simulink subsystem "Swerve_Drive_sub"  (R2023b)
settings: Solver=VariableStepAuto  StartTime=0.0  StopTime=10.0  RelTol=1e-3
undefined symbols (not defined in the file): Distance_BL_x, Distance_BL_y, Distance_BR_x, Distance_BR_y, Distance_FL_x, Distance_FL_y, Distance_FR_x, Distance_FR_y
libraries: Controls_Components_lib x8, simulink_extras x1
settings Model: Creator=ander  LastModifiedBy=ander

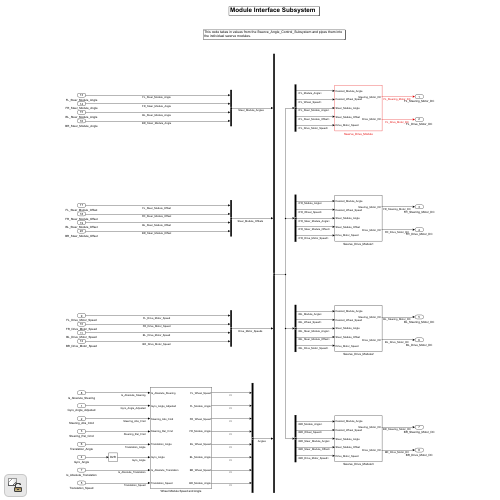
[thumbnail: Simulink's stored preview of the top-level diagram]
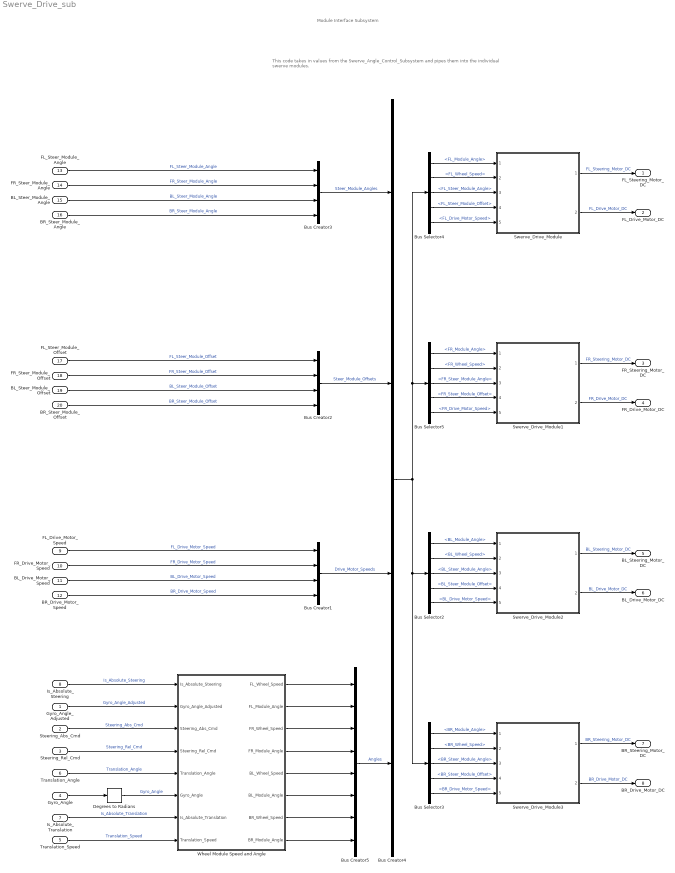
== system Swerve_Drive_sub ==
  note: This code takes in values from the Swerve_Angle_Control_Subsystem and pipes them into the individual swerve modules.
  note: Module Interface Subsystem
  Gyro_Angle_Adjusted : Inport
  Steering_Abs_Cmd : Inport  Port=2
  Steering_Rel_Cmd : Inport  Port=3
  Gyro_Angle : Inport  Port=4
  Translation_Speed : Inport  Port=5
  Translation_Angle : Inport  Port=6
  Is_Absolute_Translation : Inport  Port=7
  Is_Absolute_Steering : Inport  Port=8
  FL_Drive_Motor_Speed : Inport  Port=9
  FR_Drive_Motor_Speed : Inport  Port=10
  BL_Drive_Motor_Speed : Inport  Port=11
  BR_Drive_Motor_Speed : Inport  Port=12
  FL_Steer_Module_Angle : Inport  Port=13
  FR_Steer_Module_Angle : Inport  Port=14
  BL_Steer_Module_Angle : Inport  Port=15
  BR_Steer_Module_Angle : Inport  Port=16
  FL_Steer_Module_Offset : Inport  Port=17
  FR_Steer_Module_Offset : Inport  Port=18
  BL_Steer_Module_Offset : Inport  Port=19
  BR_Steer_Module_Offset : Inport  Port=20
  Bus Creator{1..4} (4 alike) : BusCreator  Inputs=4
  Bus Creator5 : BusCreator  Inputs=8
  Bus Selector2 : BusSelector  OutputSignals=Angles.BL_Module_Angle,Angles.BL_Wheel_Speed,Steer_Module_Angles.BL_Steer_Module_Angle,Steer_Module_Offsets.BL_Steer_Module_Offset,Drive_Motor_Speeds.BL_Drive_Motor_Speed
  Bus Selector3 : BusSelector  OutputSignals=Angles.BR_Module_Angle,Angles.BR_Wheel_Speed,Steer_Module_Angles.BR_Steer_Module_Angle,Steer_Module_Offsets.BR_Steer_Module_Offset,Drive_Motor_Speeds.BR_Drive_Motor_Speed
  Bus Selector4 : BusSelector  OutputSignals=Angles.FL_Module_Angle,Angles.FL_Wheel_Speed,Steer_Module_Angles.FL_Steer_Module_Angle,Steer_Module_Offsets.FL_Steer_Module_Offset,Drive_Motor_Speeds.FL_Drive_Motor_Speed
  Bus Selector5 : BusSelector  OutputSignals=Angles.FR_Module_Angle,Angles.FR_Wheel_Speed,Steer_Module_Angles.FR_Steer_Module_Angle,Steer_Module_Offsets.FR_Steer_Module_Offset,Drive_Motor_Speeds.FR_Drive_Motor_Speed
  Degrees to Radians : simulink_extras/Transformations/Degrees to Radians
  Swerve_Drive_Module{,1..3} (4 alike) : Subsystem  ReferencedSubsystem=Swerve_Drive_Module_sub
  Wheel Module Speed and Angle : Subsystem
  FL_Steering_Motor_DC : Outport
  FL_Drive_Motor_DC : Outport  Port=2
  FR_Steering_Motor_DC : Outport  Port=3
  FR_Drive_Motor_DC : Outport  Port=4
  BL_Steering_Motor_DC : Outport  Port=5
  BL_Drive_Motor_DC : Outport  Port=6
  BR_Steering_Motor_DC : Outport  Port=7
  BR_Drive_Motor_DC : Outport  Port=8
  wires:
  Swerve_Drive_Module/1 -> FL_Steering_Motor_DC/1  "FL_Steering_Motor_DC"
  Swerve_Drive_Module2/2 -> BL_Drive_Motor_DC/1  "BL_Drive_Motor_DC"
  Swerve_Drive_Module1/1 -> FR_Steering_Motor_DC/1  "FR_Steering_Motor_DC"
  Swerve_Drive_Module3/2 -> BR_Drive_Motor_DC/1  "BR_Drive_Motor_DC"
  Swerve_Drive_Module3/1 -> BR_Steering_Motor_DC/1  "BR_Steering_Motor_DC"
  Swerve_Drive_Module1/2 -> FR_Drive_Motor_DC/1  "FR_Drive_Motor_DC"
  Swerve_Drive_Module2/1 -> BL_Steering_Motor_DC/1  "BL_Steering_Motor_DC"
  Swerve_Drive_Module/2 -> FL_Drive_Motor_DC/1  "FL_Drive_Motor_DC"
  Bus Selector3/5 -> Swerve_Drive_Module3/5  "<BR_Drive_Motor_Speed>"
  Bus Selector3/4 -> Swerve_Drive_Module3/4  "<BR_Steer_Module_Offset>"
  Bus Selector3/2 -> Swerve_Drive_Module3/2  "<BR_Wheel_Speed>"
  Bus Selector3/3 -> Swerve_Drive_Module3/3  "<BR_Steer_Module_Angle>"
  Bus Selector3/1 -> Swerve_Drive_Module3/1  "<BR_Module_Angle>"
  Bus Selector2/5 -> Swerve_Drive_Module2/5  "<BL_Drive_Motor_Speed>"
  Bus Selector2/4 -> Swerve_Drive_Module2/4  "<BL_Steer_Module_Offset>"
  Bus Selector2/3 -> Swerve_Drive_Module2/3  "<BL_Steer_Module_Angle>"
  Bus Selector2/2 -> Swerve_Drive_Module2/2  "<BL_Wheel_Speed>"
  Bus Selector2/1 -> Swerve_Drive_Module2/1  "<BL_Module_Angle>"
  Bus Selector5/5 -> Swerve_Drive_Module1/5  "<FR_Drive_Motor_Speed>"
  Bus Selector5/4 -> Swerve_Drive_Module1/4  "<FR_Steer_Module_Offset>"
  Bus Selector5/3 -> Swerve_Drive_Module1/3  "<FR_Steer_Module_Angle>"
  Bus Selector5/2 -> Swerve_Drive_Module1/2  "<FR_Wheel_Speed>"
  Bus Selector5/1 -> Swerve_Drive_Module1/1  "<FR_Module_Angle>"
  Bus Selector4/5 -> Swerve_Drive_Module/5  "<FL_Drive_Motor_Speed>"
  Bus Selector4/4 -> Swerve_Drive_Module/4  "<FL_Steer_Module_Offset>"
  Bus Selector4/3 -> Swerve_Drive_Module/3  "<FL_Steer_Module_Angle>"
  Bus Selector4/2 -> Swerve_Drive_Module/2  "<FL_Wheel_Speed>"
  Bus Selector4/1 -> Swerve_Drive_Module/1  "<FL_Module_Angle>"
  Bus Creator4/1 -> Bus Selector3/1, Bus Selector2/1, Bus Selector4/1, Bus Selector5/1
  Bus Creator3/1 -> Bus Creator4/1  "Steer_Module_Angles"
  Bus Creator2/1 -> Bus Creator4/2  "Steer_Module_Offsets"
  Bus Creator1/1 -> Bus Creator4/3  "Drive_Motor_Speeds"
  Bus Creator5/1 -> Bus Creator4/4  "Angles"
  BR_Steer_Module_Angle/1 -> Bus Creator3/4  "BR_Steer_Module_Angle"
  BL_Steer_Module_Angle/1 -> Bus Creator3/3  "BL_Steer_Module_Angle"
  FR_Steer_Module_Angle/1 -> Bus Creator3/2  "FR_Steer_Module_Angle"
  FL_Steer_Module_Angle/1 -> Bus Creator3/1  "FL_Steer_Module_Angle"
  FL_Steer_Module_Offset/1 -> Bus Creator2/1  "FL_Steer_Module_Offset"
  FR_Steer_Module_Offset/1 -> Bus Creator2/2  "FR_Steer_Module_Offset"
  BL_Steer_Module_Offset/1 -> Bus Creator2/3  "BL_Steer_Module_Offset"
  BR_Steer_Module_Offset/1 -> Bus Creator2/4  "BR_Steer_Module_Offset"
  FL_Drive_Motor_Speed/1 -> Bus Creator1/1  "FL_Drive_Motor_Speed"
  FR_Drive_Motor_Speed/1 -> Bus Creator1/2  "FR_Drive_Motor_Speed"
  BL_Drive_Motor_Speed/1 -> Bus Creator1/3  "BL_Drive_Motor_Speed"
  BR_Drive_Motor_Speed/1 -> Bus Creator1/4  "BR_Drive_Motor_Speed"
  Is_Absolute_Steering/1 -> Wheel Module Speed and Angle/1(Is_Absolute_Steering)  "Is_Absolute_Steering"
  Gyro_Angle_Adjusted/1 -> Wheel Module Speed and Angle/2(Gyro_Angle_Adjusted)  "Gyro_Angle_Adjusted"
  Steering_Abs_Cmd/1 -> Wheel Module Speed and Angle/3(Steering_Abs_Cmd)  "Steering_Abs_Cmd"
  Steering_Rel_Cmd/1 -> Wheel Module Speed and Angle/4(Steering_Rel_Cmd)  "Steering_Rel_Cmd"
  Translation_Angle/1 -> Wheel Module Speed and Angle/5(Translation_Angle)  "Translation_Angle"
  Gyro_Angle/1 -> Degrees to Radians/1
  Is_Absolute_Translation/1 -> Wheel Module Speed and Angle/7(Is_Absolute_Translation)  "Is_Absolute_Translation"
  Translation_Speed/1 -> Wheel Module Speed and Angle/8(Translation_Speed)  "Translation_Speed"
  Wheel Module Speed and Angle/1(FL_Wheel_Speed) -> Bus Creator5/1
  Wheel Module Speed and Angle/2(FL_Module_Angle) -> Bus Creator5/2
  Wheel Module Speed and Angle/3(FR_Wheel_Speed) -> Bus Creator5/3
  Wheel Module Speed and Angle/4(FR_Module_Angle) -> Bus Creator5/4
  Wheel Module Speed and Angle/5(BL_Wheel_Speed) -> Bus Creator5/5
  Wheel Module Speed and Angle/6(BL_Module_Angle) -> Bus Creator5/6
  Wheel Module Speed and Angle/7(BR_Wheel_Speed) -> Bus Creator5/7
  Wheel Module Speed and Angle/8(BR_Module_Angle) -> Bus Creator5/8
  Degrees to Radians/1 -> Wheel Module Speed and Angle/6(Gyro_Angle)  "Gyro_Angle"

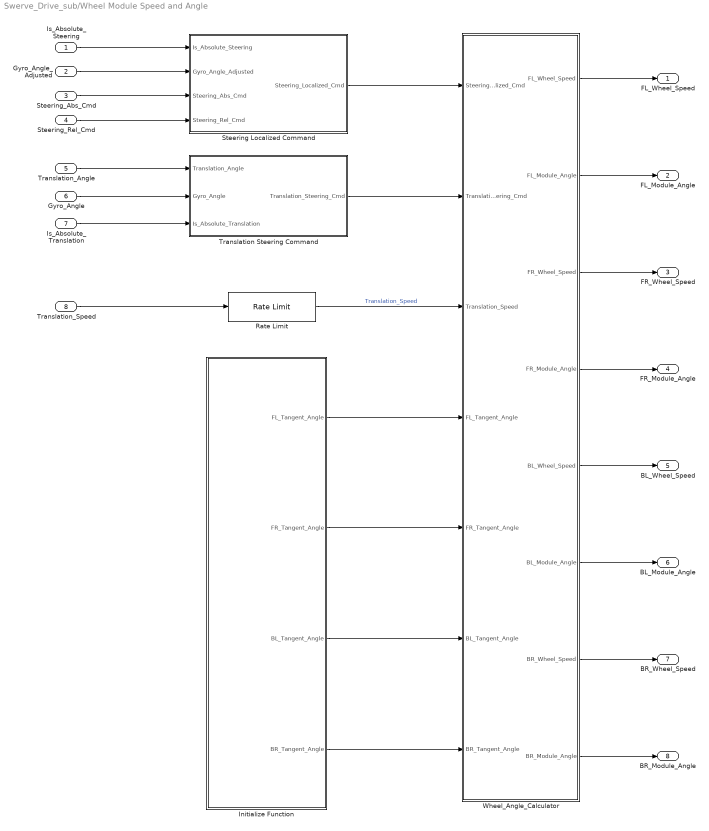
== system Swerve_Drive_sub/Wheel Module Speed and Angle ==
  Is_Absolute_Steering : Inport
  Gyro_Angle_Adjusted : Inport  Port=2
  Steering_Abs_Cmd : Inport  Port=3
  Steering_Rel_Cmd : Inport  Port=4
  Translation_Angle : Inport  Port=5
  Gyro_Angle : Inport  Port=6
  Is_Absolute_Translation : Inport  Port=7
  Translation_Speed : Inport  Port=8
  Initialize Function : Subsystem  TreatAsAtomicUnit=on
  Rate Limit : Controls_Components_lib/Rate Limit  Rate_Limit_Inc=Translation_Speed_Rate_Limit_Inc  Rate_Limit_Dec=Translation_Speed_Rate_Limit_Dec  Approaching_Zero_Error_Threshold=Translation_Speed_Approach_Zero_Error_Thresh  Approaching_Zero_Final_Scale_Factor=Translation_Speed_Approach_Zero_Final_Thresh  Approaching_NonZero_Error_Threshold=Translation_Speed_NonZero_Error_Thresh  Approaching_NonZero_Final_Scale_Factor=Translation_Speed_NonZero_Final_Scale_Factor
  Steering Localized Command : Subsystem
  Translation Steering Command : Subsystem
  Wheel_Angle_Calculator : Subsystem
  FL_Wheel_Speed : Outport
  FL_Module_Angle : Outport  Port=2
  FR_Wheel_Speed : Outport  Port=3
  FR_Module_Angle : Outport  Port=4
  BL_Wheel_Speed : Outport  Port=5
  BL_Module_Angle : Outport  Port=6
  BR_Wheel_Speed : Outport  Port=7
  BR_Module_Angle : Outport  Port=8
  wires:
  Rate Limit/1 -> Wheel_Angle_Calculator/3(Translation_Speed)  "Translation_Speed"
  Translation_Speed/1 -> Rate Limit/1
  Is_Absolute_Steering/1 -> Steering Localized Command/1(Is_Absolute_Steering)
  Gyro_Angle_Adjusted/1 -> Steering Localized Command/2(Gyro_Angle_Adjusted)
  Steering_Rel_Cmd/1 -> Steering Localized Command/4(Steering_Rel_Cmd)
  Wheel_Angle_Calculator/2(FL_Module_Angle) -> FL_Module_Angle/1
  Wheel_Angle_Calculator/4(FR_Module_Angle) -> FR_Module_Angle/1
  Wheel_Angle_Calculator/6(BL_Module_Angle) -> BL_Module_Angle/1
  Steering Localized Command/1(Steering_Localized_Cmd) -> Wheel_Angle_Calculator/1(Steering_Localized_Cmd)
  Wheel_Angle_Calculator/3(FR_Wheel_Speed) -> FR_Wheel_Speed/1
  Wheel_Angle_Calculator/1(FL_Wheel_Speed) -> FL_Wheel_Speed/1
  Wheel_Angle_Calculator/7(BR_Wheel_Speed) -> BR_Wheel_Speed/1
  Is_Absolute_Translation/1 -> Translation Steering Command/3(Is_Absolute_Translation)
  Initialize Function/4(BR_Tangent_Angle) -> Wheel_Angle_Calculator/7(BR_Tangent_Angle)
  Initialize Function/2(FR_Tangent_Angle) -> Wheel_Angle_Calculator/5(FR_Tangent_Angle)
  Wheel_Angle_Calculator/8(BR_Module_Angle) -> BR_Module_Angle/1
  Initialize Function/3(BL_Tangent_Angle) -> Wheel_Angle_Calculator/6(BL_Tangent_Angle)
  Steering_Abs_Cmd/1 -> Steering Localized Command/3(Steering_Abs_Cmd)
  Wheel_Angle_Calculator/5(BL_Wheel_Speed) -> BL_Wheel_Speed/1
  Gyro_Angle/1 -> Translation Steering Command/2(Gyro_Angle)
  Initialize Function/1(FL_Tangent_Angle) -> Wheel_Angle_Calculator/4(FL_Tangent_Angle)
  Translation Steering Command/1(Translation_Steering_Cmd) -> Wheel_Angle_Calculator/2(Translation_Steering_Cmd)
  Translation_Angle/1 -> Translation Steering Command/1(Translation_Angle)

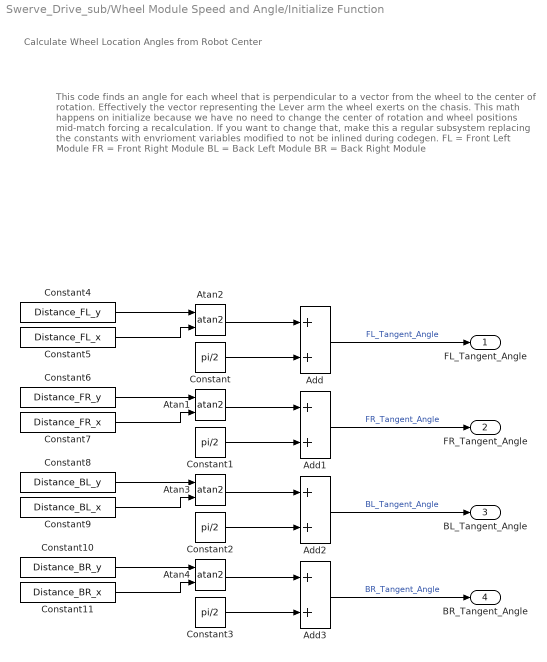
== system Swerve_Drive_sub/Wheel Module Speed and Angle/Initialize Function ==
  note: This code finds an angle for each wheel that is perpendicular to a vector from the wheel to the center of rotation. Effectively the vector representing the Lever arm the wheel exerts on the chasis. This math happens on initialize because we have no need to change the center of rotation and wheel positions mid-match forcing a recalculation. If you want to change that, make this a regular subsystem replacing the constants with envrioment variables modified to not be inlined during codegen.
      | FL = Front Left Module
      | FR = Front Right Module
      | BL = Back Left Module
      | BR = Back Right Module
  note: Calculate Wheel Location Angles from Robot Center
  Add{,1..3} (4 alike) : Sum
  Atan{1..4} (4 alike) : Trigonometry  Operator=atan2
  Constant{,1..3} (4 alike) : Constant  Value=pi/2
  Constant10 : Constant  Value=Distance_BR_y
  Constant11 : Constant  Value=Distance_BR_x
  Constant4 : Constant  Value=Distance_FL_y
  Constant5 : Constant  Value=Distance_FL_x
  Constant6 : Constant  Value=Distance_FR_y
  Constant7 : Constant  Value=Distance_FR_x
  Constant8 : Constant  Value=Distance_BL_y
  Constant9 : Constant  Value=Distance_BL_x
  FL_Tangent_Angle : Outport
  FR_Tangent_Angle : Outport  Port=2
  BL_Tangent_Angle : Outport  Port=3
  BR_Tangent_Angle : Outport  Port=4
  wires:
  Constant11/1 -> Atan4/2
  Constant10/1 -> Atan4/1
  Constant9/1 -> Atan3/2
  Constant8/1 -> Atan3/1
  Constant7/1 -> Atan1/2
  Constant6/1 -> Atan1/1
  Constant5/1 -> Atan2/2
  Constant4/1 -> Atan2/1
  Atan4/1 -> Add3/1
  Constant3/1 -> Add3/2
  Constant2/1 -> Add2/2
  Atan3/1 -> Add2/1
  Atan1/1 -> Add1/1
  Constant1/1 -> Add1/2
  Constant/1 -> Add/2
  Atan2/1 -> Add/1
  Add/1 -> FL_Tangent_Angle/1  "FL_Tangent_Angle"
  Add1/1 -> FR_Tangent_Angle/1  "FR_Tangent_Angle"
  Add2/1 -> BL_Tangent_Angle/1  "BL_Tangent_Angle"
  Add3/1 -> BR_Tangent_Angle/1  "BR_Tangent_Angle"

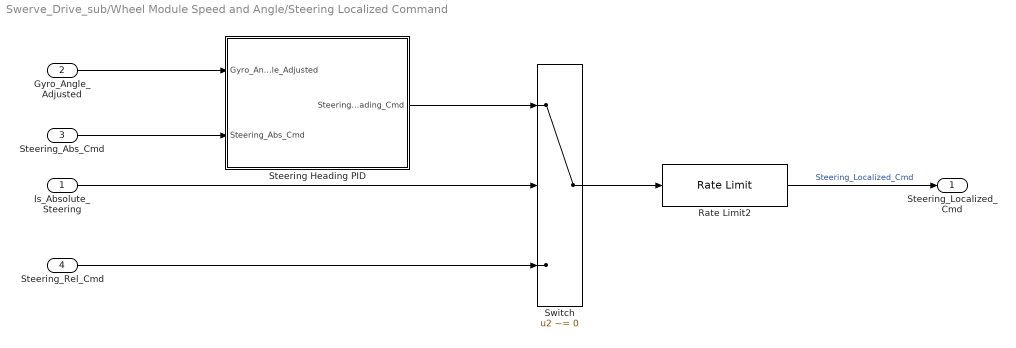
== system Swerve_Drive_sub/Wheel Module Speed and Angle/Steering Localized Command ==
  Is_Absolute_Steering : Inport
  Gyro_Angle_Adjusted : Inport  Port=2
  Steering_Abs_Cmd : Inport  Port=3
  Steering_Rel_Cmd : Inport  Port=4
  Rate Limit2 : Controls_Components_lib/Rate Limit  Rate_Limit_Inc=Steering_Localized_Cmd_Rate_Limit_Inc  Rate_Limit_Dec=Steering_Localized_Cmd_Rate_Limit_Dec  Approaching_Zero_Error_Threshold=Steering_Localized_Cmd_Approach_Zero_Error_Thresh  Approaching_Zero_Final_Scale_Factor=Steering_Localized_Cmd_Approach_Zero_Final_Thresh  Approaching_NonZero_Error_Threshold=Steering_Localized_Cmd_NonZero_Error_Thresh  Approaching_NonZero_Final_Scale_Factor=Steering_Localized_Cmd_NonZero_Final_Scale_Factor
  Steering Heading PID : Subsystem
  Switch : Switch  Criteria=u2 ~= 0  SaturateOnIntegerOverflow=off  InputSameDT=off
  Steering_Localized_Cmd : Outport
  wires:
  Rate Limit2/1 -> Steering_Localized_Cmd/1  "Steering_Localized_Cmd"
  Gyro_Angle_Adjusted/1 -> Steering Heading PID/1(Gyro_Angle_Adjusted)
  Steering_Rel_Cmd/1 -> Switch/3
  Switch/1 -> Rate Limit2/1
  Steering Heading PID/1(Steering_Heading_Cmd) -> Switch/1
  Is_Absolute_Steering/1 -> Switch/2
  Steering_Abs_Cmd/1 -> Steering Heading PID/2(Steering_Abs_Cmd)

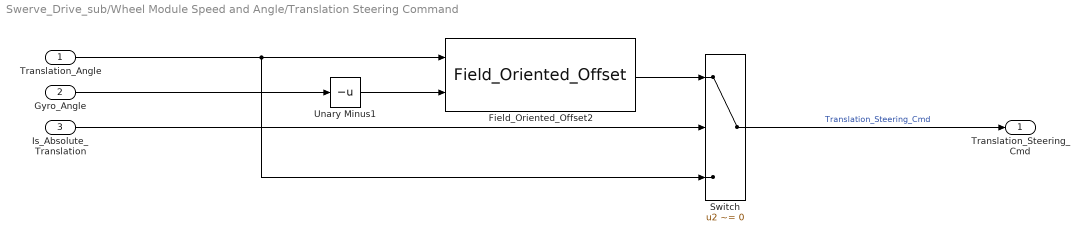
== system Swerve_Drive_sub/Wheel Module Speed and Angle/Translation Steering Command ==
  Translation_Angle : Inport
  Gyro_Angle : Inport  Port=2
  Is_Absolute_Translation : Inport  Port=3
  Field_Oriented_Offset2 : Controls_Components_lib/Field_Oriented_Offset  SystemSampleTime=-1  VariantActivationTime=update diagram  AllowFlexibleInterface=on  Latency=0  AutoFrameSizeCalculation=off
  Switch : Switch  Criteria=u2 ~= 0  SaturateOnIntegerOverflow=off  InputSameDT=off
  Unary Minus1 : UnaryMinus
  Translation_Steering_Cmd : Outport
  wires:
  Translation_Angle/1 -> Field_Oriented_Offset2/1, Switch/3
  Unary Minus1/1 -> Field_Oriented_Offset2/2
  Field_Oriented_Offset2/1 -> Switch/1
  Switch/1 -> Translation_Steering_Cmd/1  "Translation_Steering_Cmd"
  Gyro_Angle/1 -> Unary Minus1/1
  Is_Absolute_Translation/1 -> Switch/2

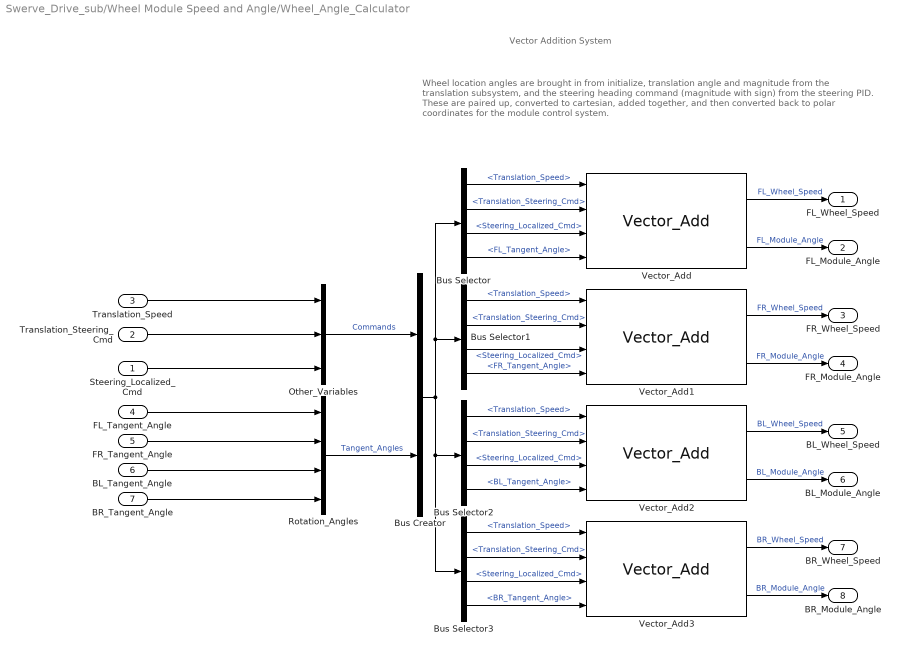
== system Swerve_Drive_sub/Wheel Module Speed and Angle/Wheel_Angle_Calculator ==
  note: Wheel location angles are brought in from initialize, translation angle and magnitude from the translation subsystem, and the steering heading command (magnitude with sign) from the steering PID. These are paired up, converted to cartesian, added together, and then converted back to polar coordinates for the module control system.
  note: Vector Addition System
  Steering_Localized_Cmd : Inport
  Translation_Steering_Cmd : Inport  Port=2
  Translation_Speed : Inport  Port=3
  FL_Tangent_Angle : Inport  Port=4
  FR_Tangent_Angle : Inport  Port=5
  BL_Tangent_Angle : Inport  Port=6
  BR_Tangent_Angle : Inport  Port=7
  Bus Creator : BusCreator  Inputs=2
  Bus Selector : BusSelector  OutputSignals=Commands.Translation_Speed,Commands.Translation_Steering_Cmd,Commands.Steering_Localized_Cmd,Tangent_Angles.FL_Tangent_Angle
  Bus Selector1 : BusSelector  OutputSignals=Commands.Translation_Speed,Commands.Translation_Steering_Cmd,Commands.Steering_Localized_Cmd,Tangent_Angles.FR_Tangent_Angle
  Bus Selector2 : BusSelector  OutputSignals=Commands.Translation_Speed,Commands.Translation_Steering_Cmd,Commands.Steering_Localized_Cmd,Tangent_Angles.BL_Tangent_Angle
  Bus Selector3 : BusSelector  OutputSignals=Commands.Translation_Speed,Commands.Translation_Steering_Cmd,Commands.Steering_Localized_Cmd,Tangent_Angles.BR_Tangent_Angle
  Other_Variables : BusCreator  Inputs=3
  Rotation_Angles : BusCreator  Inputs=4
  Vector_Add{,1..3} (4 alike) : Controls_Components_lib/Vector_Add  SystemSampleTime=-1  VariantActivationTime=update diagram  AllowFlexibleInterface=on  Latency=0  AutoFrameSizeCalculation=off
  FL_Wheel_Speed : Outport
  FL_Module_Angle : Outport  Port=2
  FR_Wheel_Speed : Outport  Port=3
  FR_Module_Angle : Outport  Port=4
  BL_Wheel_Speed : Outport  Port=5
  BL_Module_Angle : Outport  Port=6
  BR_Wheel_Speed : Outport  Port=7
  BR_Module_Angle : Outport  Port=8
  wires:
  Steering_Localized_Cmd/1 -> Other_Variables/3
  Translation_Steering_Cmd/1 -> Other_Variables/2
  Translation_Speed/1 -> Other_Variables/1
  FR_Tangent_Angle/1 -> Rotation_Angles/2
  FL_Tangent_Angle/1 -> Rotation_Angles/1
  BL_Tangent_Angle/1 -> Rotation_Angles/3
  BR_Tangent_Angle/1 -> Rotation_Angles/4
  Other_Variables/1 -> Bus Creator/1  "Commands"
  Rotation_Angles/1 -> Bus Creator/2  "Tangent_Angles"
  Bus Creator/1 -> Bus Selector/1, Bus Selector1/1, Bus Selector3/1, Bus Selector2/1
  Bus Selector/2 -> Vector_Add/2  "<Translation_Steering_Cmd>"
  Bus Selector/1 -> Vector_Add/1  "<Translation_Speed>"
  Bus Selector/3 -> Vector_Add/3  "<Steering_Localized_Cmd>"
  Bus Selector/4 -> Vector_Add/4  "<FL_Tangent_Angle>"
  Bus Selector1/1 -> Vector_Add1/1  "<Translation_Speed>"
  Bus Selector1/2 -> Vector_Add1/2  "<Translation_Steering_Cmd>"
  Bus Selector1/3 -> Vector_Add1/3  "<Steering_Localized_Cmd>"
  Bus Selector1/4 -> Vector_Add1/4  "<FR_Tangent_Angle>"
  Bus Selector2/1 -> Vector_Add2/1  "<Translation_Speed>"
  Bus Selector2/2 -> Vector_Add2/2  "<Translation_Steering_Cmd>"
  Bus Selector2/3 -> Vector_Add2/3  "<Steering_Localized_Cmd>"
  Bus Selector2/4 -> Vector_Add2/4  "<BL_Tangent_Angle>"
  Bus Selector3/1 -> Vector_Add3/1  "<Translation_Speed>"
  Bus Selector3/2 -> Vector_Add3/2  "<Translation_Steering_Cmd>"
  Bus Selector3/3 -> Vector_Add3/3  "<Steering_Localized_Cmd>"
  Bus Selector3/4 -> Vector_Add3/4  "<BR_Tangent_Angle>"
  Vector_Add/1 -> FL_Wheel_Speed/1  "FL_Wheel_Speed"
  Vector_Add/2 -> FL_Module_Angle/1  "FL_Module_Angle"
  Vector_Add1/1 -> FR_Wheel_Speed/1  "FR_Wheel_Speed"
  Vector_Add1/2 -> FR_Module_Angle/1  "FR_Module_Angle"
  Vector_Add2/1 -> BL_Wheel_Speed/1  "BL_Wheel_Speed"
  Vector_Add2/2 -> BL_Module_Angle/1  "BL_Module_Angle"
  Vector_Add3/1 -> BR_Wheel_Speed/1  "BR_Wheel_Speed"
  Vector_Add3/2 -> BR_Module_Angle/1  "BR_Module_Angle"

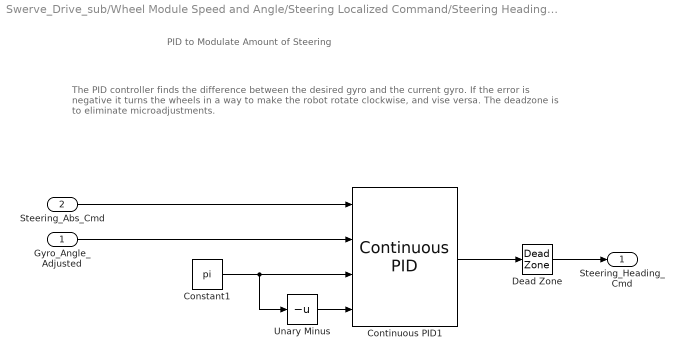
== system Swerve_Drive_sub/Wheel Module Speed and Angle/Steering Localized Command/Steering Heading PID ==
  note: PID to Modulate Amount of Steering
  note: The PID controller finds the difference between the desired gyro and the current gyro. If the error is negative it turns the wheels in a way to make the robot rotate clockwise, and vise versa.
      |
      | The deadzone is to eliminate microadjustments.
  Gyro_Angle_Adjusted : Inport
  Steering_Abs_Cmd : Inport  Port=2
  Constant1 : Constant  Value=pi
  Continuous PID1 : Controls_Components_lib/Continuous PID  Gain_P=Steering_Heading_Control_P  Gain_I=Steering_Heading_Control_I  Gain_D=Steering_Heading_Control_D  FilterCoeff_D=Steering_Heading_Control_D_FilterCoeff  Limit_I_Upper=Steering_Heading_Control_I_UL  Limit_I_Lower=Steering_Heading_Control_I_LL  Limit_D_Upper=Steering_Heading_Control_D_UL  Limit_D_Lower=Steering_Heading_Control_D_LL  Limit_T_Upper=Steering_Heading_Control_Total_UL  Limit_T_Lower=Steering_Heading_Control_Total_LL
  Dead Zone : DeadZone  LowerValue=Steering_Heading_Control_Deadzone_Neg  UpperValue=Steering_Heading_Control_Deadzone_Pos
  Unary Minus : UnaryMinus
  Steering_Heading_Cmd : Outport
  wires:
  Continuous PID1/1 -> Dead Zone/1
  Unary Minus/1 -> Continuous PID1/4
  Constant1/1 -> Continuous PID1/3, Unary Minus/1
  Steering_Abs_Cmd/1 -> Continuous PID1/1
  Gyro_Angle_Adjusted/1 -> Continuous PID1/2
  Dead Zone/1 -> Steering_Heading_Cmd/1
